simulink model "quest2"  (R2015b)
settings: Solver=ode3  StartTime=0.0  StopTime=30  FixedStep=0.01  RelTol=1e-3
values from neighbouring files (symbols this model uses):
  Kpx = 5    [staticInit.m]
  Kpy = 5    [staticInit.m]
  L = 0.13    [staticInit.m]
  r = 0.1    [staticInit.m]
  R = 2    [staticInit.m]
  wd = 0.5    [staticInit.m]
undefined symbols (not defined in the file or in its folder): F_invW
libraries: simulink x2
settings Model: Creator=smishra  LastModifiedBy=Subodh
settings DataIOCC: SaveFormat=Array
settings HardwareCC: ProdBitPerPointer=32  ProdLargestAtomicFloat=None  ProdIntDivRoundTo=Undefined  ProdEndianess=Unspecified  ProdWordSize=32  ProdHWDeviceType=32-bit Generic
settings GRTTargetCC: GeneratePreprocessorConditionals=Disable all
settings ConfigComp: CovModelRefEnable=Off

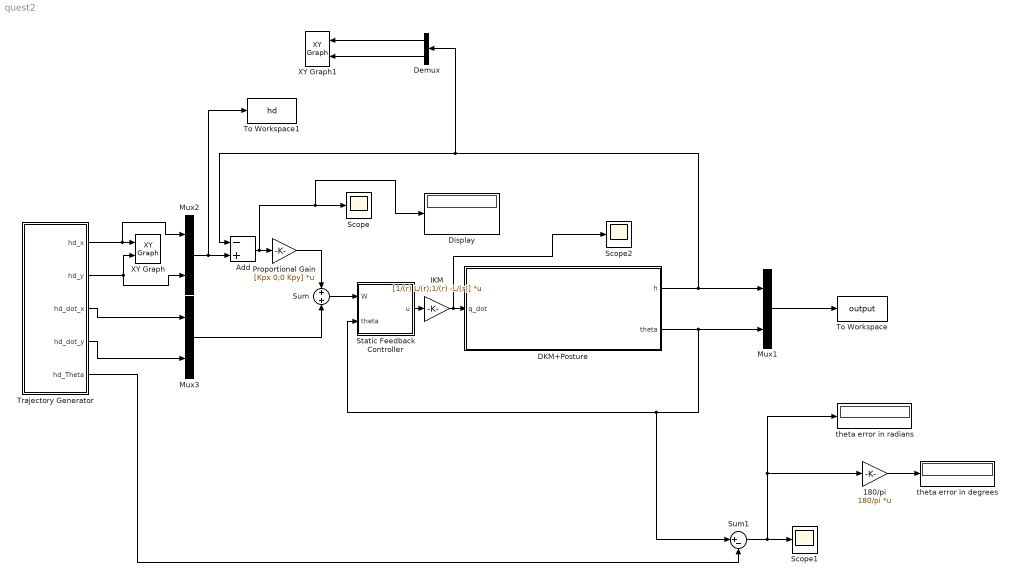
== system quest2 ==
  180/pi : Gain  Gain=180/pi  Multiplication=Matrix(K*u)
  Add : Sum  Inputs=-+
  DKM+Posture : Subsystem
  Demux : Demux  Outputs=2
  Display : Display
  IKM : Gain  Gain=[1/(r) L/(r);1/(r) -L/(r)]  Multiplication=Matrix(K*u)
  Mux1 : Mux  Inputs=2
  Mux2 : Mux  Inputs=2
  Mux3 : Mux  Inputs=2
  Proportional Gain : Gain  Gain=[Kpx 0;0 Kpy]  Multiplication=Matrix(K*u)
  Scope : Scope
  Scope1 : Scope
  Scope2 : Scope
  Static Feedback Controller : Subsystem
  Sum : Sum  Inputs=+|+
  Sum1 : Sum  Inputs=|+-
  To Workspace : ToWorkspace  VariableName=output  SampleTime=-1
  To Workspace1 : ToWorkspace  VariableName=hd  SampleTime=-1
  Trajectory Generator : Subsystem
  XY Graph : simulink/Sinks/XY Graph  xmin=-2.5  xmax=2.5  ymin=-2.5  ymax=2.5  st=-1
  XY Graph1 : simulink/Sinks/XY Graph  xmin=-2.5  xmax=2.5  ymin=-2.5  ymax=2.5  st=-1
  theta error in degrees : Display
  theta error in radians : Display
  wires:
  Trajectory Generator/1(hd_x) -> Mux2/1, XY Graph/1
  Trajectory Generator/2(hd_y) -> XY Graph/2, Mux2/2
  Trajectory Generator/3(hd_dot_x) -> Mux3/1
  Trajectory Generator/4(hd_dot_y) -> Mux3/2
  Mux2/1 -> To Workspace1/1, Add/2
  Mux3/1 -> Sum/2
  Add/1 -> Display/1, Scope/1, Proportional Gain/1
  Proportional Gain/1 -> Sum/1
  Sum/1 -> Static Feedback Controller/1(W)
  Static Feedback Controller/1(u) -> IKM/1
  IKM/1 -> Scope2/1, DKM+Posture/1(q_dot)
  Demux/1 -> XY Graph1/1
  Demux/2 -> XY Graph1/2
  DKM+Posture/1(h) -> Demux/1, Add/1, Mux1/1
  DKM+Posture/2(theta) -> Mux1/2, Sum1/1, Static Feedback Controller/2(theta)
  Mux1/1 -> To Workspace/1
  Sum1/1 -> 180/pi/1, theta error in radians/1, Scope1/1
  Trajectory Generator/5(hd_Theta) -> Sum1/2
  180/pi/1 -> theta error in degrees/1

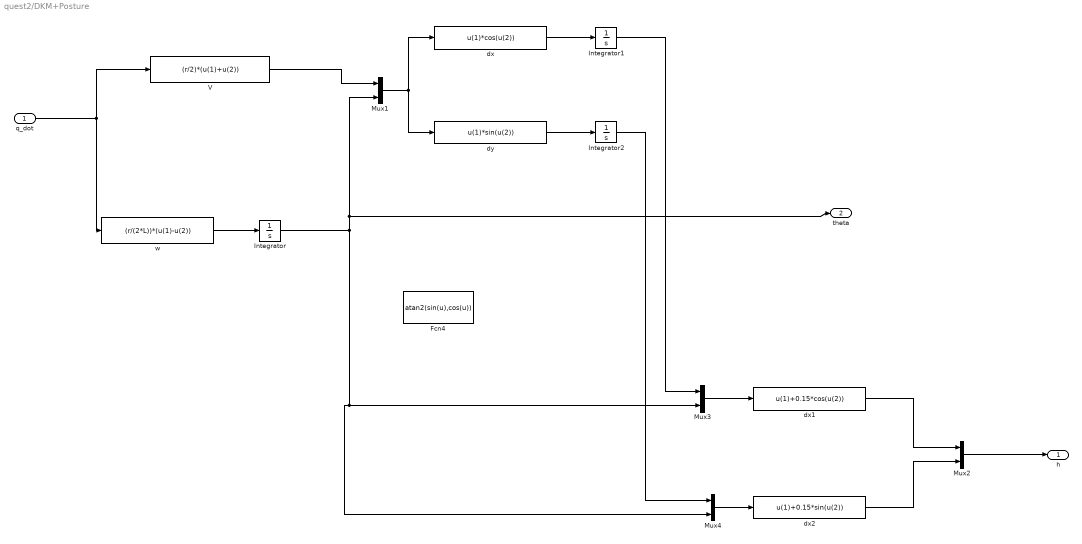
== system quest2/DKM+Posture ==
  q_dot : Inport
  Fcn4 : Fcn  Expr=atan2(sin(u),cos(u))
  Integrator : Integrator  InitialCondition=pi
  Integrator1 : Integrator  InitialCondition=2.45
  Integrator2 : Integrator
  Mux{1..4} (4 alike) : Mux  Inputs=2
  V : Fcn  Expr=(r/2)*(u(1)+u(2))
  dx : Fcn  Expr=u(1)*cos(u(2))
  dx1 : Fcn  Expr=u(1)+0.15*cos(u(2))
  dx2 : Fcn  Expr=u(1)+0.15*sin(u(2))
  dy : Fcn  Expr=u(1)*sin(u(2))
  w : Fcn  Expr=(r/(2*L))*(u(1)-u(2))
  h : Outport
  theta : Outport  Port=2
  wires:
  q_dot/1 -> V/1, w/1
  w/1 -> Integrator/1
  Integrator1/1 -> Mux3/1
  dy/1 -> Integrator2/1
  Mux1/1 -> dy/1, dx/1
  Integrator2/1 -> Mux4/1
  dx/1 -> Integrator1/1
  V/1 -> Mux1/1
  Integrator/1 -> Mux4/2, Mux3/2, Mux1/2, theta/1
  Mux2/1 -> h/1
  Mux3/1 -> dx1/1
  Mux4/1 -> dx2/1
  dx1/1 -> Mux2/1
  dx2/1 -> Mux2/2

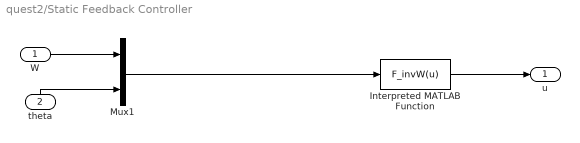
== system quest2/Static Feedback Controller ==
  W : Inport
  theta : Inport  Port=2
  Interpreted MATLAB Function : MATLABFcn  MATLABFcn=F_invW(u)  OutputDimensions=[2 1]  OutputSignalType=real  Output1D=off
  Mux1 : Mux  Inputs=2
  u : Outport
  wires:
  theta/1 -> Mux1/2
  W/1 -> Mux1/1
  Interpreted MATLAB Function/1 -> u/1
  Mux1/1 -> Interpreted MATLAB Function/1

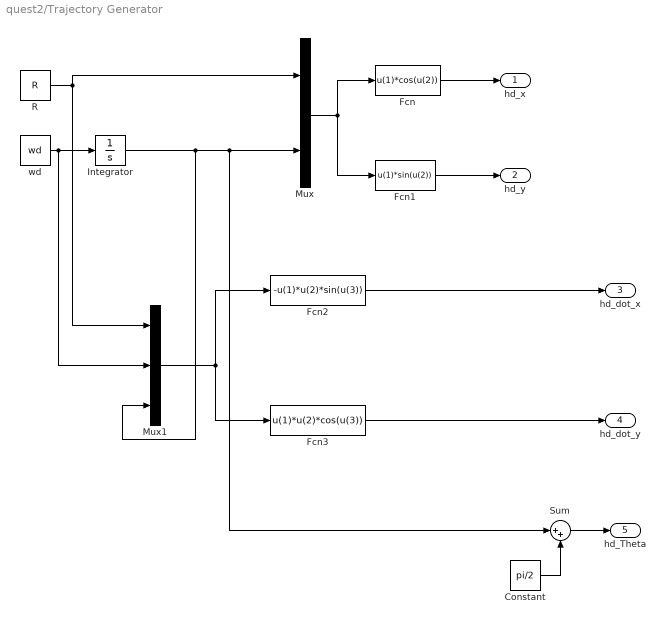
== system quest2/Trajectory Generator ==
  Constant : Constant  Value=pi/2
  Fcn : Fcn  Expr=u(1)*cos(u(2))
  Fcn1 : Fcn  Expr=u(1)*sin(u(2))
  Fcn2 : Fcn  Expr=-u(1)*u(2)*sin(u(3))
  Fcn3 : Fcn  Expr=u(1)*u(2)*cos(u(3))
  Integrator : Integrator
  Mux : Mux  Inputs=2
  Mux1 : Mux  Inputs=3
  R : Constant  Value=R
  Sum : Sum  Inputs=|++
  wd : Constant  Value=wd
  hd_x : Outport
  hd_y : Outport  Port=2
  hd_dot_x : Outport  Port=3
  hd_dot_y : Outport  Port=4
  hd_Theta : Outport  Port=5
  wires:
  Fcn/1 -> hd_x/1
  Mux1/1 -> Fcn2/1, Fcn3/1
  Fcn3/1 -> hd_dot_y/1
  Fcn1/1 -> hd_y/1
  Mux/1 -> Fcn/1, Fcn1/1
  R/1 -> Mux1/1, Mux/1
  Fcn2/1 -> hd_dot_x/1
  wd/1 -> Mux1/2, Integrator/1
  Integrator/1 -> Sum/1, Mux/2, Mux1/3
  Sum/1 -> hd_Theta/1
  Constant/1 -> Sum/2
